simulink model "Final_Model"  (R2018a)
settings: Solver=ode23tb  StartTime=0.0  StopTime=0.15  MaxStep=1e-2  RelTol=1e-3
undefined symbols (not defined in the file): rvar
libraries: powerlib x75, powerlib_extras x4, sps_avr x2, powerlib_meascontrol x1
settings Model: Creator=Mahdi  LastModifiedBy=Lenovo
settings SolverCC: ZeroCrossAlgorithm=Adaptive  SolverResetMethod=Robust
settings DataIOCC: LimitDataPoints=on  SaveFormat=Array
settings OptimizationCC: LifeSpan=inf
settings DebuggingCC: UnderspecifiedInitializationDetection=Classic  MergeDetectMultiDrivingBlocksExec=none  SolverPrmCheckMsg=warning  LibraryContextMissingDiagnostic=warning  SFUnexpectedBacktrackingDiag=warning  SFNoUnconditionalDefaultTransitionDiag=warning  SFExecutionAtInitializationDiag=none
settings HardwareCC: ProdBitPerPointer=32  ProdBitPerSizeT=32  ProdBitPerPtrDiffT=32  ProdLargestAtomicFloat=None  ProdIntDivRoundTo=Undefined  ProdEndianess=Unspecified  ProdWordSize=32  ProdHWDeviceType=32-bit Generic
settings ModelReferenceCC: PropagateSignalLabelsOutOfModel=off
settings CodeAppCC: StateflowObjectComments=on
settings GRTTargetCC: TargetLangStandard=C89/C90 (ANSI)  GeneratePreprocessorConditionals=Disable all
settings ConfigComp: CovMetricSettings=dw  CovHtmlReporting=on  CovSaveCumulativeToWorkspaceVar=on  CovSaveSingleToWorkspaceVar=on  CovExternalEMLEnable=off
settings SimscapeCC: SimscapeNormalizeSystem=off

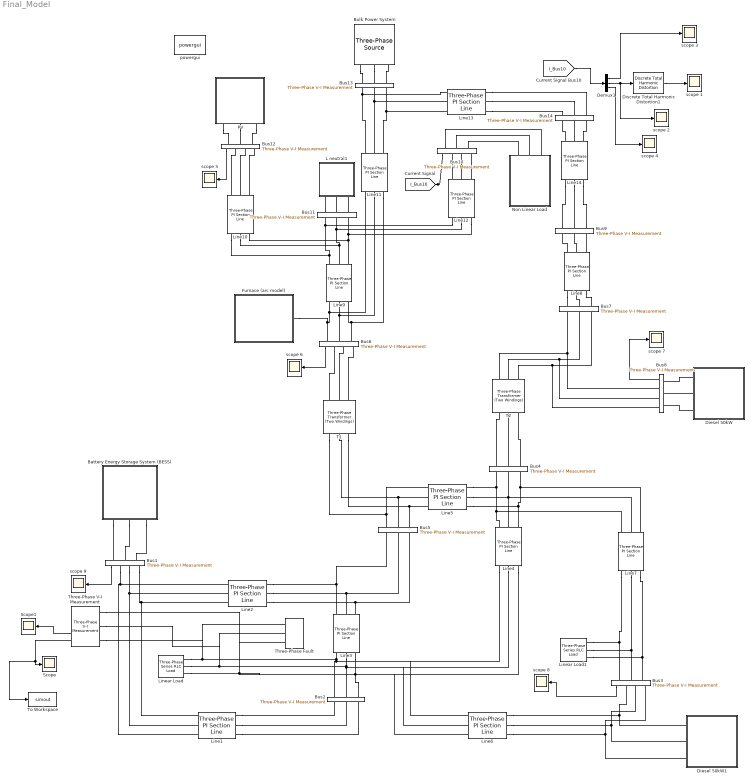
== system Final_Model ==
  " L neutral1" : Subsystem
  Battery Energy Storage System (BESS) : Subsystem
  Bulk Power System : powerlib/Electrical Sources/Three-Phase Source  InternalConnection=Yg  VoltagePhases=off  Voltage=25e3  PhaseAngle=0  Voltage_phases=[25e3 25e3 25e3]/sqrt(3)  PhaseAngles_phases=[0 -120 +120]  Frequency=60  NonIdealSource=on  SpecifyImpedance=on  Resistance=0.8929  Inductance=16.58e-3  ShortCircuitLevel=100e6  BaseVoltage=25e3  XRratio=7  BusType=swing  Pref=0  Qref=0  Prefabc=[10e3, 10e3, 10e3]  Qrefabc=[0, 0, 0]  Qmin=-inf  Qmax=inf
  Bus{1,3,6,8,10,12} (6 alike) : powerlib/Measurements/Three-Phase V-I Measurement  VoltageMeasurement=no  SetLabelV=off  LabelV=Vabc  Vpu=off  VpuLL=off  CurrentMeasurement=yes  SetLabelI=off  LabelI=Iabc  Ipu=off  Pbase=100e6  Vbase=500e3  OutputType=Complex  PhasorSimulation=off  PSBequivalent=0
  Bus{2,4..5,7,9,11,13..14} (8 alike) : powerlib/Measurements/Three-Phase V-I Measurement  VoltageMeasurement=no  SetLabelV=off  LabelV=Vabc  Vpu=off  VpuLL=off  CurrentMeasurement=no  SetLabelI=off  LabelI=Iabc  Ipu=off  Pbase=100e6  Vbase=500e3  OutputType=Complex  PhasorSimulation=off  PSBequivalent=0
  Demux1 : Demux  Outputs=3
  Diesel 50kW : Subsystem
  Diesel 50kW1 : Subsystem
  Discrete Total Harmonic Distortion1 : powerlib_extras/Discrete Measurements/Discrete Total Harmonic Distortion  Freq=50  Ts=50e-6
  Furnace (arc model) : Subsystem
  Line1 : powerlib/Elements/Three-Phase PI Section Line  LConnTagsString=a|b|c  RConnTagsString=A|B|C  Frequency=60  Resistances=[ 0.01273 0.3864]  Inductances="[ 0.9337e-3  4.1264e-3]"  Capacitances=[12.74e-9 7.751e-9]  Length=3
      settings: SourceProductName=Simscape Power Systems
  Line{2..3,6,9..10,12} (6 alike) : powerlib/Elements/Three-Phase PI Section Line  LConnTagsString=a|b|c  RConnTagsString=A|B|C  Frequency=60  Resistances=[ 0.01273 0.3864]  Inductances="[ 0.9337e-3  4.1264e-3]"  Capacitances=[12.74e-9 7.751e-9]  Length=2
      settings: SourceProductName=Simscape Power Systems
  Line11 : powerlib/Elements/Three-Phase PI Section Line  LConnTagsString=a|b|c  RConnTagsString=A|B|C  Frequency=60  Resistances=[ 0.01273 0.3864]  Inductances="[ 0.9337e-3  4.1264e-3]"  Capacitances=[12.74e-9 7.751e-9]  Length=1.5
      settings: SourceProductName=Simscape Power Systems
  Line13 : powerlib/Elements/Three-Phase PI Section Line  LConnTagsString=a|b|c  RConnTagsString=A|B|C  Frequency=60  Resistances=[ 0.01273 0.3864]  Inductances="[ 0.9337e-3  4.1264e-3]"  Capacitances=[12.74e-9 7.751e-9]  Length=1
      settings: SourceProductName=Simscape Power Systems
  Line14 : powerlib/Elements/Three-Phase PI Section Line  LConnTagsString=a|b|c  RConnTagsString=A|B|C  Frequency=60  Resistances=[ 0.01273 0.3864]  Inductances="[ 0.9337e-3  4.1264e-3]"  Capacitances=[12.74e-9 7.751e-9]  Length=1
      settings: SourceProductName=Simscape Power Systems
  Line4 : powerlib/Elements/Three-Phase PI Section Line  LConnTagsString=a|b|c  RConnTagsString=A|B|C  Frequency=60  Resistances=[ 0.01273 0.3864]  Inductances="[ 0.9337e-3  4.1264e-3]"  Capacitances=[12.74e-9 7.751e-9]  Length=3
      settings: SourceProductName=Simscape Power Systems
  Line5 : powerlib/Elements/Three-Phase PI Section Line  LConnTagsString=a|b|c  RConnTagsString=A|B|C  Frequency=60  Resistances=[ 0.01273 0.3864]  Inductances="[ 0.9337e-3  4.1264e-3]"  Capacitances=[12.74e-9 7.751e-9]  Length=3
      settings: SourceProductName=Simscape Power Systems
  Line7 : powerlib/Elements/Three-Phase PI Section Line  LConnTagsString=a|b|c  RConnTagsString=A|B|C  Frequency=60  Resistances=[ 0.01273 0.3864]  Inductances="[ 0.9337e-3  4.1264e-3]"  Capacitances=[12.74e-9 7.751e-9]  Length=2.4
      settings: SourceProductName=Simscape Power Systems
  Line8 : powerlib/Elements/Three-Phase PI Section Line  LConnTagsString=a|b|c  RConnTagsString=A|B|C  Frequency=60  Resistances=[ 0.01273 0.3864]  Inductances="[ 0.9337e-3  4.1264e-3]"  Capacitances=[12.74e-9 7.751e-9]  Length=1
      settings: SourceProductName=Simscape Power Systems
  Linear Load : powerlib/Elements/Three-Phase Series RLC Load  LConnTagsString=A|B|C  Configuration=Y (grounded)  NominalVoltage=1000  Vabc=[1e3 1e3 1e3]  Vabcp=[1e3 1e3 1e3]  NominalFrequency=60  UnbalancedPower=off  ActivePower=1e3  InductivePower=100  CapacitivePower=100  Pabc=[10e3 9e3 11e3]  QLabc=[100 90 110]  QCabc=[100 90 110]  Pabcp=[10e3 9e3 11e3]  QLabcp=[100 90 110]  QCabcp=[100 90 110]  Measurements=None  LoadType=constant Z
  Linear Load1 : powerlib/Elements/Three-Phase Series RLC Load  LConnTagsString=A|B|C  Configuration=Y (grounded)  NominalVoltage=1000  Vabc=[1e3 1e3 1e3]  Vabcp=[1e3 1e3 1e3]  NominalFrequency=60  UnbalancedPower=off  ActivePower=1e3  InductivePower=100  CapacitivePower=100  Pabc=[10e3 9e3 11e3]  QLabc=[100 90 110]  QCabc=[100 90 110]  Pabcp=[10e3 9e3 11e3]  QLabcp=[100 90 110]  QCabcp=[100 90 110]  Measurements=None  LoadType=constant Z
  Non Linear Load : Subsystem
  PV : Subsystem
  Scope : Scope
  Scope1 : Scope
  T1 : powerlib/Elements/Three-Phase Transformer (Two Windings)  Winding1Connection=Yg  Winding2Connection=Yg  CoreType=Three single-phase transformers  SetSaturation=off  Hysteresis=off  DataFile='hysteresis'  SetInitialFlux=off  Measurements=None  UNITS=pu  NominalPower=[ 250e6 , 60 ]  Winding1=[ 0.735e3 , 0.002 , 0.08 ]  Winding2=[ 255e3 , 0.002 , 0.08 ]  Rm=500  Lm=500  L0=0.5  Saturation=[ 0,0 ; 0.0024,1.2 ; 1.0,1.52 ]  InitialFluxes=[ 0.8 , -0.8 , 0.7 ]  MoreParameters=off  BreakLoop=off  DataType=off  TransfoNumber=1
  T2 : powerlib/Elements/Three-Phase Transformer (Two Windings)  Winding1Connection=Yg  Winding2Connection=Yg  CoreType=Three single-phase transformers  SetSaturation=off  Hysteresis=off  DataFile='hysteresis'  SetInitialFlux=off  Measurements=None  UNITS=pu  NominalPower=[ 250e6 , 60 ]  Winding1=[ 0.735e3 , 0.002 , 0.08 ]  Winding2=[ 25e3 , 0.002 , 0.08 ]  Rm=500  Lm=500  L0=0.5  Saturation=[ 0,0 ; 0.0024,1.2 ; 1.0,1.52 ]  InitialFluxes=[ 0.8 , -0.8 , 0.7 ]  MoreParameters=off  BreakLoop=off  DataType=off  TransfoNumber=1
  Three-Phase V-I Measurement : powerlib/Measurements/Three-Phase V-I Measurement  VoltageMeasurement=phase-to-ground  SetLabelV=off  LabelV=Vabc  Vpu=off  VpuLL=off  CurrentMeasurement=yes  SetLabelI=off  LabelI=Iabc  Ipu=off  Pbase=100e6  Vbase=500e3  OutputType=Complex  PhasorSimulation=off  PSBequivalent=0
  Three-Phase Fault : powerlib/Elements/Three-Phase Fault  InitialStates=0  FaultA=on  FaultB=on  FaultC=off  GroundFault=on  SwitchTimes="[0.04  0.08]"  External=off  SwitchStatus=NaN  FaultResistance=0.00001  GroundResistance=0.0001  SnubberResistance=1e6  SnubberCapacitance=inf  Measurements=None
  To Workspace : ToWorkspace  VariableName=simout  SampleTime=-1
  powergui : powerlib/powergui  Priority=1  SimulationMode=Discrete  SampleTime=2e-5  frequency=60  Iterations=50  frequencyindice=0  Pbase=100e6  ErrMax=1e-4  UnitsV=kV  UnitsW=MW  buscounter=0  FunctionMessages=off  echomessages=off  EnableUseOfTLC=off  CurrentSourceSwitches=off  DisableSnubberDevices=off  DisableRonSwitches=off  DisableVfSwitches=off  DisplayEquations=off  SolverType=Tustin  Interpol=off  ExternalGateDelay=off  methode=off  Ts=0  x0status=blocks  SPID=off  SwTol=0  HookPort=off  RestoreLinks=warning  ResistiveCurrentMeasurement=off  Frange=[0:2:500]  Ylog=off  Xlog=on  ShowGrid=off  save=off  variable=ZData  structure=0  ZoomFFT=off  StartTime=0.0  cycles=1  DisplayStyle=1  fundamental=60  FreqAxis=off  MaxFrequency=1000  frequencyindicesteady=1  RmsSteady=1  display=off
  scope {1..9} (9 alike) : Scope
  tag scope: I_Bus10=global
  wires:
  [I_Bus10] -> Demux1/1
  Discrete Total Harmonic Distortion1/1 -> scope 1/1
  Bus10/1 -> [I_Bus10]
  Demux1/2 -> scope 2/1, Discrete Total Harmonic Distortion1/1
  Demux1/1 -> scope 3/1
  Demux1/3 -> scope 4/1
  Bus12/1 -> scope 5/1
  Bus6/1 -> scope 6/1
  Bus8/1 -> scope 7/1
  Bus3/1 -> scope 8/1
  Bus1/1 -> scope 9/1
  Three-Phase V-I Measurement/1 -> To Workspace/1, Scope/1
  Three-Phase V-I Measurement/2 -> Scope1/1
  connections:
  Bus1/RConn1 -- Line1/LConn3 -- Line2/LConn1
  Bus1/RConn2 -- Line1/LConn2 -- Line2/LConn2
  Bus1/RConn3 -- Line1/LConn1 -- Line2/LConn3
  Line1/RConn1 -- Bus2/RConn1
  Line1/RConn2 -- Bus2/RConn2
  Line1/RConn3 -- Bus2/RConn3
  Line2/RConn1 -- Line3/RConn1 -- Bus5/RConn1
  Line2/RConn2 -- Line3/RConn2 -- Bus5/RConn2
  Line2/RConn3 -- Line3/RConn3 -- Bus5/RConn3
  Line3/LConn1 -- Three-Phase Fault/LConn1 -- Three-Phase V-I Measurement/LConn1 -- Linear Load/LConn1 -- Bus2/LConn1 -- Line6/LConn1 -- Line4/LConn1
  Line3/LConn2 -- Three-Phase Fault/LConn2 -- Three-Phase V-I Measurement/LConn2 -- Linear Load/LConn2 -- Line6/LConn2 -- Line4/LConn2 -- Bus2/LConn2
  Line3/LConn3 -- Three-Phase V-I Measurement/LConn3 -- Three-Phase Fault/LConn3 -- Linear Load/LConn3 -- Line6/LConn3 -- Line4/LConn3 -- Bus2/LConn3
  Line4/RConn1 -- Line7/RConn1 -- Bus4/RConn1 -- Line5/RConn1
  Line4/RConn2 -- Line7/RConn2 -- Bus4/RConn2 -- Line5/RConn2
  Line4/RConn3 -- Line5/RConn3 -- Line7/RConn3 -- Bus4/RConn3
  Line5/LConn1 -- T1/LConn1 -- Bus5/LConn1
  Line5/LConn2 -- Bus5/LConn2 -- T1/LConn2
  Line5/LConn3 -- T1/LConn3 -- Bus5/LConn3
  Line6/RConn1 -- Bus3/RConn1 -- Diesel 50kW1/LConn1
  Line6/RConn2 -- Bus3/RConn2 -- Diesel 50kW1/LConn2
  Line6/RConn3 -- Bus3/RConn3 -- Diesel 50kW1/LConn3
  Line7/LConn1 -- Bus3/LConn1 -- Linear Load1/LConn1
  Line7/LConn2 -- Bus3/LConn2 -- Linear Load1/LConn2
  Line7/LConn3 -- Bus3/LConn3 -- Linear Load1/LConn3
  Line8/LConn1 -- Bus7/LConn1
  Bus7/LConn2 -- Line8/LConn2
  Line8/LConn3 -- Bus7/LConn3
  Line8/RConn1 -- Bus9/RConn1
  Line8/RConn2 -- Bus9/RConn2
  Line8/RConn3 -- Bus9/RConn3
  Bus12/RConn1 -- Line10/RConn1
  Bus12/RConn2 -- Line10/RConn2
  Bus12/RConn3 -- Line10/RConn3
  Bus6/LConn1 -- Furnace (arc model)/LConn1 -- Line11/LConn1 -- Line9/LConn1
  Bus6/LConn2 -- Line11/LConn2 -- Line9/LConn2
  Bus6/LConn3 -- Line9/LConn3 -- Line11/LConn3
  Line9/RConn1 -- Line10/LConn1 -- Line12/LConn1 -- Bus11/RConn1
  Line9/RConn2 -- Line10/LConn2 -- Line12/LConn2 -- Bus11/RConn2
  Line9/RConn3 -- Line10/LConn3 -- Line12/LConn3 -- Bus11/RConn3
  Line11/RConn1 -- Line13/LConn1 -- Bus13/RConn1
  Line11/RConn2 -- Bus13/RConn2 -- Line13/LConn2
  Line11/RConn3 -- Bus13/RConn3 -- Line13/LConn3
  Line12/RConn1 -- Bus10/RConn1
  Line12/RConn2 -- Bus10/RConn2
  Line12/RConn3 -- Bus10/RConn3
  Line13/RConn1 -- Bus14/LConn3
  Line13/RConn2 -- Bus14/LConn2
  Line13/RConn3 -- Bus14/LConn1
  Line14/RConn3 -- Bus14/RConn3
  Line14/RConn2 -- Bus14/RConn2
  Line14/RConn1 -- Bus14/RConn1
  Line14/LConn3 -- Bus9/LConn3
  Line14/LConn2 -- Bus9/LConn2
  Line14/LConn1 -- Bus9/LConn1
  T1/RConn1 -- Bus6/RConn1
  T1/RConn2 -- Bus6/RConn2
  T1/RConn3 -- Bus6/RConn3
  Bus4/LConn1 -- T2/LConn1
  Bus4/LConn2 -- T2/LConn2
  Bus4/LConn3 -- T2/LConn3
  T2/RConn1 -- Bus8/RConn1 -- Bus7/RConn1
  T2/RConn2 -- Bus8/RConn2 -- Bus7/RConn2
  T2/RConn3 -- Bus8/RConn3 -- Bus7/RConn3
  Diesel 50kW/LConn1 -- Bus8/LConn1
  Diesel 50kW/LConn2 -- Bus8/LConn2
  Diesel 50kW/LConn3 -- Bus8/LConn3
  Battery Energy Storage System (BESS)/LConn1 -- Bus1/LConn1
  Battery Energy Storage System (BESS)/LConn2 -- Bus1/LConn2
  Battery Energy Storage System (BESS)/LConn3 -- Bus1/LConn3
  PV/LConn1 -- Bus12/LConn1
  PV/LConn2 -- Bus12/LConn2
  PV/LConn3 -- Bus12/LConn3
  Bus11/LConn1 -- " L neutral1"/LConn1
  Bus11/LConn2 -- " L neutral1"/LConn2
  Bus11/LConn3 -- " L neutral1"/LConn3
  Non Linear Load/LConn1 -- Bus10/LConn3
  Non Linear Load/LConn2 -- Bus10/LConn2
  Non Linear Load/LConn3 -- Bus10/LConn1
  Bulk Power System/RConn1 -- Bus13/LConn1
  Bulk Power System/RConn2 -- Bus13/LConn2
  Bulk Power System/RConn3 -- Bus13/LConn3

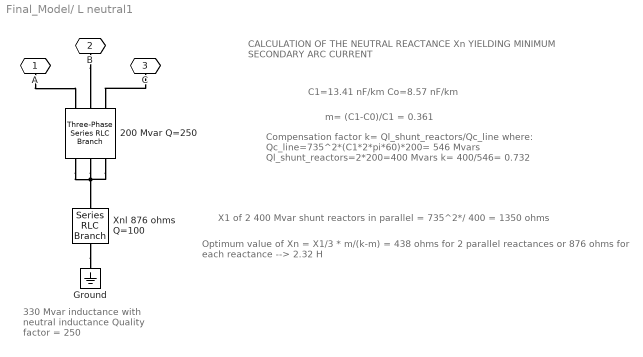
== system Final_Model/ L neutral1 ==
  note: CALCULATION OF THE NEUTRAL REACTANCE Xn
      | YIELDING MINIMUM SECONDARY ARC CURRENT
  note: X1 of 2 400 Mvar shunt reactors in parallel = 735^2*/ 400 = 1350 ohms
  note: Optimum value of Xn = X1/3 * m/(k-m) = 438 ohms for 2 parallel reactances
      | or 876 ohms for each reactance --> 2.32 H
  note: Compensation factor k= Ql_shunt_reactors/Qc_line
      | where:
      |  Qc_line=735^2*(C1*2*pi*60)*200= 546 Mvars
      |  Ql_shunt_reactors=2*200=400 Mvars
      | k= 400/546= 0.732
  note: m= (C1-C0)/C1 = 0.361
  note: C1=13.41 nF/km Co=8.57 nF/km
  note: 330 Mvar inductance
      | with neutral inductance
      | Quality factor = 250
  200 Mvar Q=250 : powerlib/Elements/Three-Phase Series RLC Branch  LConnTagsString=A|B|C  RConnTagsString=A|B|C  BranchType=RL  Resistance=735^2/200/250  Inductance=.735^2/.200/.377  Capacitance=1.0  Measurements=None
  Ground : powerlib/Elements/Ground  LConnTagsString=a
  Xnl 876 ohms Q=100 : powerlib/Elements/Series RLC Branch  LConnTagsString=__new0  RConnTagsString=__new0  BranchType=RL  Resistance=876/100  Inductance=8.76/377  SetiL0=off  InitialCurrent=0  Capacitance=1.0  Setx0=off  InitialVoltage=0  Measurements=None
  A : PMIOPort  Side=Left
  B : PMIOPort  Port=2  Side=Left
  C : PMIOPort  Port=3  Side=Left
  connections:
  A/RConn1 -- 200 Mvar Q=250/LConn1
  B/RConn1 -- 200 Mvar Q=250/LConn2
  C/RConn1 -- 200 Mvar Q=250/LConn3
  200 Mvar Q=250/RConn3 -- 200 Mvar Q=250/RConn2 -- Xnl 876 ohms Q=100/LConn1 -- 200 Mvar Q=250/RConn1
  Xnl 876 ohms Q=100/RConn1 -- Ground/LConn1

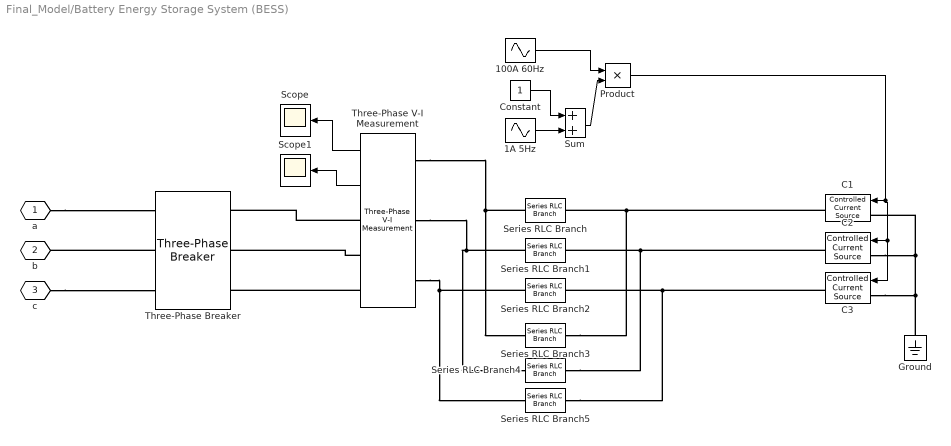
== system Final_Model/Battery Energy Storage System (BESS) ==
  100A 60Hz : Sin  Amplitude=100  Frequency=2*pi*60  SampleTime=0
  1A 5Hz : Sin  Frequency=2*pi*5  SampleTime=0
  C1 : powerlib/Electrical Sources/Controlled Current Source  Initialize=on  Source_Type=AC  Amplitude=0  Phase=0  Frequency=0  Measurements=None
  C2 : powerlib/Electrical Sources/Controlled Current Source  Initialize=on  Source_Type=AC  Amplitude=0  Phase=0  Frequency=0  Measurements=None
  C3 : powerlib/Electrical Sources/Controlled Current Source  Initialize=on  Source_Type=AC  Amplitude=0  Phase=0  Frequency=0  Measurements=None
  Constant : Constant
  Ground : powerlib/Elements/Ground  LConnTagsString=a
  Product : Product  SaturateOnIntegerOverflow=on  InputSameDT=on  OutDataTypeStr=Inherit: Same as first input
  Scope : Scope
  Scope1 : Scope
  Series RLC Branch : powerlib/Elements/Series RLC Branch  LConnTagsString=__new0  RConnTagsString=__new0  BranchType=L  Resistance=1  Inductance=1e-3  SetiL0=off  InitialCurrent=0  Capacitance=1e-6  Setx0=off  InitialVoltage=0  Measurements=None
  Series RLC Branch1 : powerlib/Elements/Series RLC Branch  LConnTagsString=__new0  RConnTagsString=__new0  BranchType=L  Resistance=1  Inductance=1e-3  SetiL0=off  InitialCurrent=0  Capacitance=1e-6  Setx0=off  InitialVoltage=0  Measurements=None
  Series RLC Branch2 : powerlib/Elements/Series RLC Branch  LConnTagsString=__new0  RConnTagsString=__new0  BranchType=L  Resistance=1  Inductance=1e-3  SetiL0=off  InitialCurrent=0  Capacitance=1e-6  Setx0=off  InitialVoltage=0  Measurements=None
  Series RLC Branch3 : powerlib/Elements/Series RLC Branch  LConnTagsString=__new0  RConnTagsString=__new0  BranchType=R  Resistance=1  Inductance=1e-3  SetiL0=off  InitialCurrent=0  Capacitance=1e-6  Setx0=off  InitialVoltage=0  Measurements=None
  Series RLC Branch4 : powerlib/Elements/Series RLC Branch  LConnTagsString=__new0  RConnTagsString=__new0  BranchType=R  Resistance=1  Inductance=1e-3  SetiL0=off  InitialCurrent=0  Capacitance=1e-6  Setx0=off  InitialVoltage=0  Measurements=None
  Series RLC Branch5 : powerlib/Elements/Series RLC Branch  LConnTagsString=__new0  RConnTagsString=__new0  BranchType=R  Resistance=1  Inductance=1e-3  SetiL0=off  InitialCurrent=0  Capacitance=1e-6  Setx0=off  InitialVoltage=0  Measurements=None
  Sum : Sum  SaturateOnIntegerOverflow=on  InputSameDT=on  OutDataTypeStr=Inherit: Same as first input
  Three-Phase V-I Measurement : powerlib/Measurements/Three-Phase V-I Measurement  VoltageMeasurement=phase-to-ground  SetLabelV=off  LabelV=Vabc  Vpu=off  VpuLL=off  CurrentMeasurement=yes  SetLabelI=off  LabelI=Iabc  Ipu=off  Pbase=100e6  Vbase=500e3  OutputType=Complex  PhasorSimulation=off  PSBequivalent=0
  Three-Phase Breaker : powerlib/Elements/Three-Phase Breaker  InitialState=closed  SwitchA=on  SwitchB=on  SwitchC=on  SwitchTimes="[4/60  10/60]"  External=off  BreakerResistance=0.001  SnubberResistance=1e6  SnubberCapacitance=inf  Measurements=None
  "a " : PMIOPort  Tag=PMCPort  Side=Left
  b : PMIOPort  Tag=PMCPort  Port=2  Side=Left
  c : PMIOPort  Tag=PMCPort  Port=3  Side=Left
  wires:
  1A 5Hz/1 -> Sum/2
  Constant/1 -> Sum/1
  Sum/1 -> Product/2
  100A 60Hz/1 -> Product/1
  Three-Phase V-I Measurement/1 -> Scope/1
  Three-Phase V-I Measurement/2 -> Scope1/1
  Product/1 -> C3/1, C2/1, C1/1
  connections:
  c/RConn1 -- Three-Phase Breaker/LConn3
  "a "/RConn1 -- Three-Phase Breaker/LConn1
  Series RLC Branch1/LConn1 -- Three-Phase V-I Measurement/LConn2 -- Series RLC Branch4/LConn1
  Series RLC Branch/LConn1 -- Series RLC Branch3/LConn1 -- Three-Phase V-I Measurement/LConn1
  Series RLC Branch2/LConn1 -- Three-Phase V-I Measurement/LConn3 -- Series RLC Branch5/LConn1
  C1/RConn1 -- Series RLC Branch3/RConn1 -- Series RLC Branch/RConn1
  C2/RConn1 -- Series RLC Branch4/RConn1 -- Series RLC Branch1/RConn1
  C3/RConn1 -- Series RLC Branch5/RConn1 -- Series RLC Branch2/RConn1
  Ground/LConn1 -- C3/LConn1 -- C2/LConn1 -- C1/LConn1
  Three-Phase Breaker/LConn2 -- b/RConn1
  Three-Phase V-I Measurement/RConn3 -- Three-Phase Breaker/RConn3
  Three-Phase V-I Measurement/RConn2 -- Three-Phase Breaker/RConn2
  Three-Phase V-I Measurement/RConn1 -- Three-Phase Breaker/RConn1

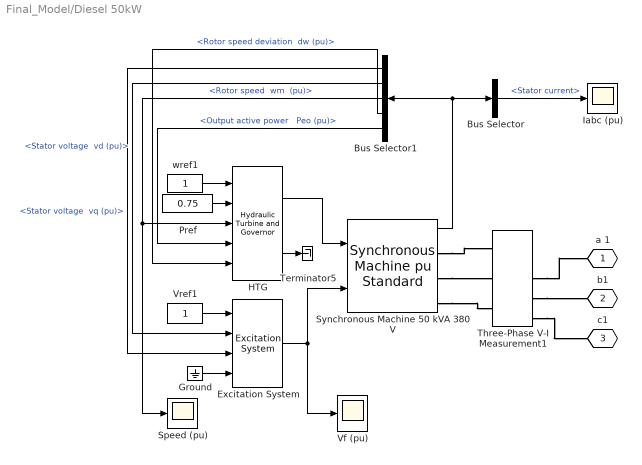
== system Final_Model/Diesel 50kW ==
  " Iabc (pu)" : Scope
  " Speed (pu)" : Scope
  Bus Selector : BusSelector  OutputSignals=Stator current
  Bus Selector1 : BusSelector  OutputSignals="dq0 components.Stator voltage  vq (pu),dq0 components.Stator voltage  vd (pu),Mechanical.Rotor speed  wm  (pu),Mechanical.Rotor speed deviation  dw (pu),Output active power   Peo (pu)"
  Excitation System : sps_avr/Excitation System  tr=20e-3  reg=[ 300, 0.001 ]  exc=[ 1, 0 ]  tgr=[ 0, 0 ]  damp=[ 0.001, 0.1 ]  sat=[ 0, 0 ]  lim=[ -11.5, 11.5, 0 ]  v0=[1,1.29071]
      settings: SourceProductName=Simscape Power Systems  SourceProductBaseCode=PS
  Ground : Ground
  HTG : powerlib/Machines/Hydraulic Turbine and Governor  sm="[ 10/3  0.07 ]"  gate="[  0.01  0.97518  -0.1  0.1 ]"  reg="[  0.05  1.163  0.105  0  0.01  ]"  hyd="[  0  2.67  ]"  dref=0  po=0.751606
      settings: SourceProductName=Simscape Power Systems  SourceProductBaseCode=PS
  Pref : Constant  Value=0.75
  Synchronous Machine 50 kVA 380 V : powerlib/Machines/Synchronous Machine pu Standard  PresetModel=No  MechanicalLoad=Mechanical power Pm  ShowDetailedParameters=on  RotorType=Salient-pole  Units=per unit standard parameters  MeasurementBus=off  NominalParameters="[ 50E3  380   60 ]"  Reactances1=[ 31 32 33 34 35 36 37 ]  Reactances2=[ 1.305, 0.296, 0.252, 0.474, 0.243, 0.18 ]  dAxisTimeConstants=Short-circuit  qAxisTimeConstants=Open-circuit  TimeConstants1=[]  TimeConstants2=[]  TimeConstants3=[]  TimeConstants4=[]  TimeConstants5=[ 1.01, 0.053, 0.1 ]  TimeConstants6=[]  TimeConstants7=[]  TimeConstants8=[]  StatorResistance=2.8544e-3  Mechanical=[ 3.2 0 2]  PolePairs=2  InitialConditions=[0 -94.2826 0.750185 0.750185 0.750185 -24.943 -144.943 95.057 1.29071]  SetSaturation=off  Saturation=[0.6404,0.7127,0.8441,0.9214,0.9956,1.082,1.19,1.316,1.457;0.7,0.7698,0.8872,0.9466,0.9969,1.046,1.1,1.151,1.201]  LoadFlowParameters=[1 150000000 0 0]  TsPowergui=0  TsBlock=-1  IterativeModel=Trapezoidal iterative (alg. loop)  IterativeDiscreteModel=Trapezoidal non iterative  BusType=PV  Pref=150000000  Qref=0  Qmin=-Inf  Qmax=Inf  PLF=0  QLF=0
      settings: AttributesFormatString=\n\n  SourceProductName=Simscape Power Systems
  Terminator5 : Terminator
  Three-Phase V-I Measurement1 : powerlib/Measurements/Three-Phase V-I Measurement  VoltageMeasurement=phase-to-ground  SetLabelV=off  LabelV=Vabc  Vpu=off  VpuLL=off  CurrentMeasurement=yes  SetLabelI=off  LabelI=Iabc  Ipu=off  Pbase=100e6  Vbase=500e3  OutputType=Complex  PhasorSimulation=off  PSBequivalent=0
  Vf (pu) : Scope
  Vref1 : Constant
  wref1 : Constant
  a 1 : PMIOPort  Tag=PMCPort  Side=Left
  b1 : PMIOPort  Tag=PMCPort  Port=2  Side=Left
  c1 : PMIOPort  Tag=PMCPort  Port=3  Side=Left
  wires:
  Ground/1 -> Excitation System/4
  HTG/2 -> Terminator5/1
  Pref/1 -> HTG/2
  Excitation System/1 -> Vf (pu)/1, Synchronous Machine 50 kVA 380 V/2
  HTG/1 -> Synchronous Machine 50 kVA 380 V/1
  Synchronous Machine 50 kVA 380 V/1 -> Bus Selector/1, Bus Selector1/1
  Bus Selector/1 -> " Iabc (pu)"/1  "<Stator current>"
  Bus Selector1/1 -> Excitation System/3  "<Stator voltage  vq (pu)>"
  Bus Selector1/2 -> Excitation System/2  "<Stator voltage  vd (pu)>"
  Bus Selector1/3 -> HTG/3, " Speed (pu)"/1  "<Rotor speed  wm  (pu)>"
  Bus Selector1/4 -> HTG/5  "<Rotor speed deviation  dw (pu)>"
  Bus Selector1/5 -> HTG/4  "<Output active power   Peo (pu)>"
  Vref1/1 -> Excitation System/1
  wref1/1 -> HTG/1
  connections:
  Synchronous Machine 50 kVA 380 V/RConn1 -- Three-Phase V-I Measurement1/LConn1
  Synchronous Machine 50 kVA 380 V/RConn2 -- Three-Phase V-I Measurement1/LConn2
  Synchronous Machine 50 kVA 380 V/RConn3 -- Three-Phase V-I Measurement1/LConn3
  Three-Phase V-I Measurement1/RConn1 -- a 1/RConn1
  Three-Phase V-I Measurement1/RConn2 -- b1/RConn1
  Three-Phase V-I Measurement1/RConn3 -- c1/RConn1

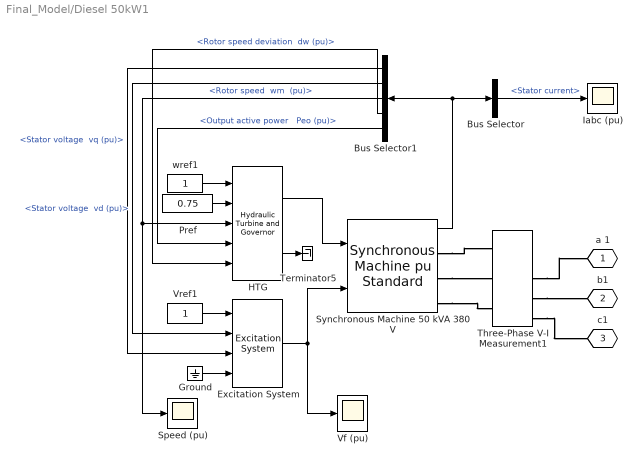
== system Final_Model/Diesel 50kW1 ==
  " Iabc (pu)" : Scope
  " Speed (pu)" : Scope
  Bus Selector : BusSelector  OutputSignals=Stator current
  Bus Selector1 : BusSelector  OutputSignals="dq0 components.Stator voltage  vq (pu),dq0 components.Stator voltage  vd (pu),Mechanical.Rotor speed  wm  (pu),Mechanical.Rotor speed deviation  dw (pu),Output active power   Peo (pu)"
  Excitation System : sps_avr/Excitation System  tr=20e-3  reg=[ 300, 0.001 ]  exc=[ 1, 0 ]  tgr=[ 0, 0 ]  damp=[ 0.001, 0.1 ]  sat=[ 0, 0 ]  lim=[ -11.5, 11.5, 0 ]  v0=[1,1.29071]
      settings: SourceProductName=Simscape Power Systems  SourceProductBaseCode=PS
  Ground : Ground
  HTG : powerlib/Machines/Hydraulic Turbine and Governor  sm="[ 10/3  0.07 ]"  gate="[  0.01  0.97518  -0.1  0.1 ]"  reg="[  0.05  1.163  0.105  0  0.01  ]"  hyd="[  0  2.67  ]"  dref=0  po=0.751606
      settings: SourceProductName=Simscape Power Systems  SourceProductBaseCode=PS
  Pref : Constant  Value=0.75
  Synchronous Machine 50 kVA 380 V : powerlib/Machines/Synchronous Machine pu Standard  PresetModel=No  MechanicalLoad=Mechanical power Pm  ShowDetailedParameters=on  RotorType=Salient-pole  Units=per unit standard parameters  MeasurementBus=off  NominalParameters="[ 50E3  380   60 ]"  Reactances1=[ 31 32 33 34 35 36 37 ]  Reactances2=[ 1.305, 0.296, 0.252, 0.474, 0.243, 0.18 ]  dAxisTimeConstants=Short-circuit  qAxisTimeConstants=Open-circuit  TimeConstants1=[]  TimeConstants2=[]  TimeConstants3=[]  TimeConstants4=[]  TimeConstants5=[ 1.01, 0.053, 0.1 ]  TimeConstants6=[]  TimeConstants7=[]  TimeConstants8=[]  StatorResistance=2.8544e-3  Mechanical=[ 3.2 0 2]  PolePairs=2  InitialConditions=[0 -94.2826 0.750185 0.750185 0.750185 -24.943 -144.943 95.057 1.29071]  SetSaturation=off  Saturation=[0.6404,0.7127,0.8441,0.9214,0.9956,1.082,1.19,1.316,1.457;0.7,0.7698,0.8872,0.9466,0.9969,1.046,1.1,1.151,1.201]  LoadFlowParameters=[1 150000000 0 0]  TsPowergui=0  TsBlock=-1  IterativeModel=Trapezoidal iterative (alg. loop)  IterativeDiscreteModel=Trapezoidal non iterative  BusType=PV  Pref=150000000  Qref=0  Qmin=-Inf  Qmax=Inf  PLF=0  QLF=0
      settings: AttributesFormatString=\n\n  SourceProductName=Simscape Power Systems
  Terminator5 : Terminator
  Three-Phase V-I Measurement1 : powerlib/Measurements/Three-Phase V-I Measurement  VoltageMeasurement=phase-to-ground  SetLabelV=off  LabelV=Vabc  Vpu=off  VpuLL=off  CurrentMeasurement=yes  SetLabelI=off  LabelI=Iabc  Ipu=off  Pbase=100e6  Vbase=500e3  OutputType=Complex  PhasorSimulation=off  PSBequivalent=0
  Vf (pu) : Scope
  Vref1 : Constant
  wref1 : Constant
  a 1 : PMIOPort  Tag=PMCPort  Side=Left
  b1 : PMIOPort  Tag=PMCPort  Port=2  Side=Left
  c1 : PMIOPort  Tag=PMCPort  Port=3  Side=Left
  wires:
  wref1/1 -> HTG/1
  Vref1/1 -> Excitation System/1
  Bus Selector1/5 -> HTG/4  "<Output active power   Peo (pu)>"
  Bus Selector1/4 -> HTG/5  "<Rotor speed deviation  dw (pu)>"
  Bus Selector1/3 -> " Speed (pu)"/1, HTG/3  "<Rotor speed  wm  (pu)>"
  Bus Selector1/2 -> Excitation System/2  "<Stator voltage  vd (pu)>"
  Bus Selector1/1 -> Excitation System/3  "<Stator voltage  vq (pu)>"
  Bus Selector/1 -> " Iabc (pu)"/1  "<Stator current>"
  Synchronous Machine 50 kVA 380 V/1 -> Bus Selector1/1, Bus Selector/1
  HTG/1 -> Synchronous Machine 50 kVA 380 V/1
  Excitation System/1 -> Synchronous Machine 50 kVA 380 V/2, Vf (pu)/1
  Pref/1 -> HTG/2
  HTG/2 -> Terminator5/1
  Ground/1 -> Excitation System/4
  connections:
  Three-Phase V-I Measurement1/RConn3 -- c1/RConn1
  Three-Phase V-I Measurement1/RConn2 -- b1/RConn1
  Three-Phase V-I Measurement1/RConn1 -- a 1/RConn1
  Synchronous Machine 50 kVA 380 V/RConn3 -- Three-Phase V-I Measurement1/LConn3
  Synchronous Machine 50 kVA 380 V/RConn2 -- Three-Phase V-I Measurement1/LConn2
  Synchronous Machine 50 kVA 380 V/RConn1 -- Three-Phase V-I Measurement1/LConn1

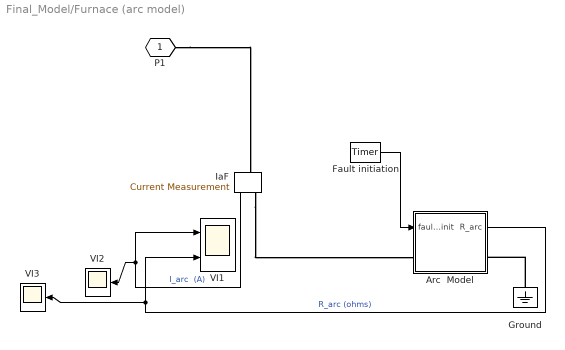
== system Final_Model/Furnace (arc model) ==
  Arc  Model : Subsystem  mask(Arc model){Rarc_var=on, Rarc_fixed=0.1, Rparam=[56.54 0.006375], I0=50, Ts=50e-6}
      mask prompts: Rarc_var "Variable arc resistance :"; Rarc_fixed "Arc resistance for fixed arc resistance :"; Rparam "Arc parameters for variable arc resistance [Ro k] : :"; I0 "Current threshold for arc extinction Io (A rms) :"; Ts "Sample time (s) :"
      mask help:
      | This block implements a variable or fixed arc resistance model.
      |
      | Input 1, output 1:  Connection terminals of the arc resistance.
      | Input 2 :    Control signal for the fault initiation
      | Use a short pulse of 1 cycle. Once fault current starts flowing, it is sustained by the arc ionized path.
      | Output 2:  Arc resitance
      |
      | If you check the 'Variable arc resistance' box, the mean arc resistance will be a function of the arc current, according to equation below. Otherwise, the resistance will be kept constant.
      |
      |        Rarc= Ro*exp(-k*i)
      |
      | where:   i = rms value of the arc current (A)
      |              Ro, k = arc parameters
      |
      | The arc extinguishes at the next zero current crossing after its  rms value has fallen  below  the specified threshold current Io.
      mask init:
      | if strcmp(Rarc_var,'on'), rvar=1; else, rvar=0; end
      | R0=Rparam(1);
      | k=Rparam(2);
  Fault initiation : powerlib_extras/Control  Blocks/Timer  t=[ 1/60 2/60 ]  e="[1 0  ]"
  Ground : powerlib/Elements/Ground  LConnTagsString=a
  IaF : powerlib/Measurements/Current Measurement  Tag=PoWeRsYsTeMmEaSuReMeNt  PhasorSimulation=off  OutputType=Magnitude  PSBequivalent=0
  VI1 : Scope  NumInputPorts=2
  VI2 : Scope
  VI3 : Scope
  P1 : PMIOPort  Tag=PMCPort  Side=Left
  wires:
  Fault initiation/1 -> Arc  Model/1(fault_init)
  Arc  Model/1(R_arc) -> VI1/2, VI3/1  "R_arc (ohms)"
  IaF/1 -> VI1/1, VI2/1  "I_arc  (A)"
  connections:
  Ground/LConn1 -- Arc  Model/RConn1
  IaF/RConn1 -- Arc  Model/LConn1
  P1/RConn1 -- IaF/LConn1

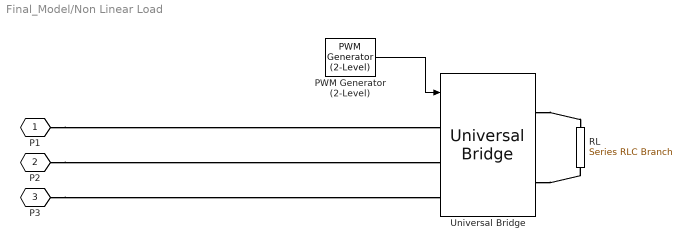
== system Final_Model/Non Linear Load ==
  PWM Generator (2-Level) : powerlib_meascontrol/Pulse & Signal Generators/PWM Generator (2-Level)  ModulatorType=Three-phase bridge (6 pulses)  ModulatorMode=Unsynchronized  Fc=4080  Pc=90  nF=27  MinMax="[ -1  1 ]"  SamplingTechnique=Natural  ModulatingSignals=on  m=0.8  Freq=60  Phase=0  Ts=0  ShowCarrierOutport=off
      settings: SourceProductName=Simscape Power Systems
  RL : powerlib/Elements/Series RLC Branch  LConnTagsString=__new0  RConnTagsString=__new0  BranchType=RL  Resistance=1  Inductance=5e-3  SetiL0=off  InitialCurrent=0  Capacitance=1e-6  Setx0=off  InitialVoltage=0  Measurements=None
  Universal Bridge : powerlib/Power Electronics/Universal Bridge  Arms=3  SnubberResistance=1e5  SnubberCapacitance=inf  Device=Thyristors  Ron=1e-3  Lon=0  ForwardVoltages="[  0  0  ]"  ForwardVoltage=0  GTOparameters=[ 10e-6 , 20e-6 ]  IGBTparameters=[ 1e-6 , 2e-6 ]  Measurements=None  Measurements_2=None  converterType=Rectifier
  P1 : PMIOPort  Tag=PMCPort  Side=Left
  P2 : PMIOPort  Tag=PMCPort  Port=2  Side=Left
  P3 : PMIOPort  Tag=PMCPort  Port=3  Side=Left
  wires:
  PWM Generator (2-Level)/1 -> Universal Bridge/1
  connections:
  Universal Bridge/RConn1 -- RL/LConn1
  P1/RConn1 -- Universal Bridge/LConn1
  P3/RConn1 -- Universal Bridge/LConn3
  P2/RConn1 -- Universal Bridge/LConn2
  Universal Bridge/RConn2 -- RL/RConn1

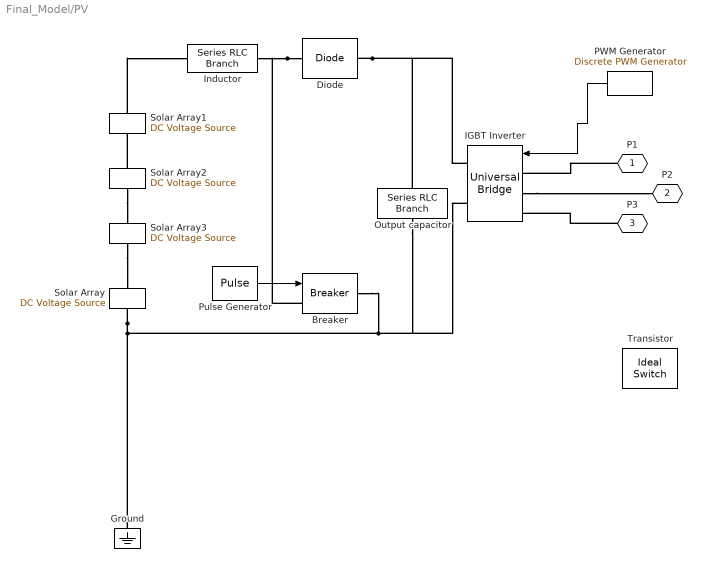
== system Final_Model/PV ==
  Breaker : powerlib/Elements/Breaker  InitialState=0  SwitchingTimes="[ 1/60  5/60 ]"  External=on  BreakerResistance=0.01  SnubberResistance=1e6  SnubberCapacitance=inf  Measurements=None  MoreParameters=off  NoBreakLoop=off
      settings: SourceProductName=Simscape Power Systems
  Diode : powerlib/Power Electronics/Diode  Ron=0.001  Lon=0  Vf=0.8  IC=0  UseSnubber=off  Rs=500  Cs=250e-9  Measurements=off
  Ground : powerlib/Elements/Ground  LConnTagsString=a
  IGBT Inverter : powerlib/Power Electronics/Universal Bridge  Arms=3  SnubberResistance=1e5  SnubberCapacitance=inf  Device=IGBT / Diodes  Ron=1e-3  Lon=0  ForwardVoltages="[  0  0  ]"  ForwardVoltage=0  GTOparameters=[ 10e-6 , 20e-6 ]  IGBTparameters=[ 1e-6 , 2e-6 ]  Measurements=All voltages and currents  Measurements_2=None  converterType=Rectifier
  Inductor : powerlib/Elements/Series RLC Branch  LConnTagsString=__new0  RConnTagsString=__new0  BranchType=L  Resistance=1  Inductance=100e-3  SetiL0=off  InitialCurrent=0  Capacitance=1e-6  Setx0=off  InitialVoltage=0  Measurements=Branch current
  Output capacitor : powerlib/Elements/Series RLC Branch  LConnTagsString=__new0  RConnTagsString=__new0  BranchType=C  Resistance=1.0  Inductance=1e-3  SetiL0=off  InitialCurrent=0  Capacitance=1000e-6  Setx0=off  InitialVoltage=0  Measurements=None
  PWM Generator : powerlib_extras/Discrete  Control Blocks/Discrete PWM Generator  GeneratorMode="3-arm  bridge (6 pulses)"  Fc=900  Ts=5.14e-6  Internal=on  mIndex=0.85  Freq=50  Phase=0
  Pulse Generator : DiscretePulseGenerator  PulseType=Time based  Amplitude=5  Period=1e-6  PulseWidth=50
  Solar Array{,1..3} (4 alike) : powerlib/Electrical Sources/DC Voltage Source  Amplitude=35  Measurements=None
  Transistor : powerlib/Power Electronics/Ideal Switch  Ron=0.001  Lon=0  IC=0  Rs=1e5  Cs=inf  Measurements=on
  "P1 " : PMIOPort  Tag=PMCPort  Side=Left
  P2 : PMIOPort  Tag=PMCPort  Port=2  Side=Left
  P3 : PMIOPort  Tag=PMCPort  Port=3  Side=Left
  wires:
  PWM Generator/1 -> IGBT Inverter/1
  Pulse Generator/1 -> Breaker/1
  connections:
  Solar Array/LConn1 -- Breaker/RConn1 -- IGBT Inverter/RConn2 -- Output capacitor/RConn1 -- Ground/LConn1
  Diode/LConn1 -- Breaker/LConn1 -- Inductor/RConn1
  Diode/RConn1 -- IGBT Inverter/RConn1 -- Output capacitor/LConn1
  Solar Array3/LConn1 -- Solar Array/RConn1
  Solar Array2/RConn1 -- Solar Array1/LConn1
  "P1 "/RConn1 -- IGBT Inverter/LConn1
  P3/RConn1 -- IGBT Inverter/LConn3
  Solar Array2/LConn1 -- Solar Array3/RConn1
  Solar Array1/RConn1 -- Inductor/LConn1
  IGBT Inverter/LConn2 -- P2/RConn1

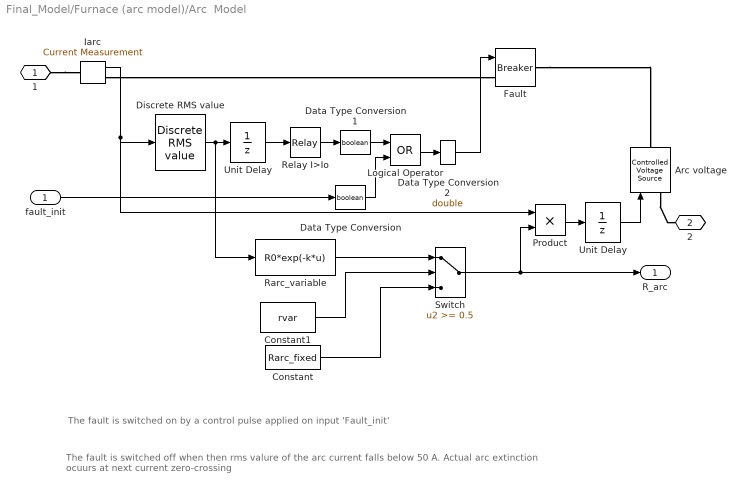
== system Final_Model/Furnace (arc model)/Arc  Model ==
  note: The fault is switched on by a control pulse applied on input 'Fault_init'
  note: The fault is switched off when then rms valure of the arc current falls below  50 A.
      | Actual arc extinction ocuurs at next current zero-crossing
  fault_init : Inport
  Arc voltage : powerlib/Electrical Sources/Controlled Voltage Source  Description=source block  Initialize=on  Source_Type=AC  Amplitude=0  Phase=0  Frequency=0  Measurements=None
      settings: AttributesFormatString=\n
  Constant : Constant  Value=Rarc_fixed
  Constant1 : Constant  Value=rvar
  Data Type Conversion : DataTypeConversion  OutDataTypeStr=boolean  SaturateOnIntegerOverflow=on  RndMeth=Zero
  Data Type Conversion1 : DataTypeConversion  OutDataTypeStr=boolean  SaturateOnIntegerOverflow=on  RndMeth=Zero
  Data Type Conversion2 : DataTypeConversion  OutDataTypeStr=double  SaturateOnIntegerOverflow=on  RndMeth=Zero
  Discrete RMS value : powerlib_extras/Discrete Measurements/Discrete  RMS value  Freq=60  Mag_Init=0  Ts=Ts
  Fault : powerlib/Elements/Breaker  InitialState=0  SwitchingTimes="[ 4/60  5/60 ]"  External=on  BreakerResistance=.001  SnubberResistance=inf  SnubberCapacitance=0  Measurements=None  MoreParameters=off  NoBreakLoop=off
      settings: AttributesFormatString=\n  SourceProductName=Simscape Power Systems
  Iarc : powerlib/Measurements/Current Measurement  Tag=PoWeRsYsTeMmEaSuReMeNt  PhasorSimulation=off  OutputType=Magnitude  PSBequivalent=0
  Logical Operator : Logic  Operator=OR
  Product : Product  SaturateOnIntegerOverflow=on  InputSameDT=on  OutDataTypeStr=Inherit: Same as first input
  Rarc_variable : Fcn  Expr=R0*exp(-k*u)
  Relay I>Io : Relay  OnSwitchValue=I0*1.2  OffSwitchValue=I0  ZeroCross=off
  Switch : Switch  Threshold=0.5  ZeroCross=off  InputSameDT=on
  Unit Delay : UnitDelay  SampleTime=Ts
  "Unit Delay " : UnitDelay  SampleTime=Ts
  1 : PMIOPort  Side=Left
  2 : PMIOPort  Port=2  Side=Right
  R_arc : Outport
  wires:
  Discrete RMS value/1 -> "Unit Delay "/1, Rarc_variable/1
  Rarc_variable/1 -> Switch/1
  Switch/1 -> Product/2, R_arc/1
  Constant/1 -> Switch/3
  Constant1/1 -> Switch/2
  Product/1 -> Unit Delay/1
  "Unit Delay "/1 -> Relay I>Io/1
  fault_init/1 -> Data Type Conversion/1
  Data Type Conversion/1 -> Logical Operator/2
  Relay I>Io/1 -> Data Type Conversion1/1
  Data Type Conversion1/1 -> Logical Operator/1
  Logical Operator/1 -> Data Type Conversion2/1
  Iarc/1 -> Product/1, Discrete RMS value/1
  Unit Delay/1 -> Arc voltage/1
  Data Type Conversion2/1 -> Fault/1
  connections:
  1/RConn1 -- Iarc/LConn1
  Iarc/RConn1 -- Fault/LConn1
  Arc voltage/LConn1 -- 2/RConn1
  Fault/RConn1 -- Arc voltage/RConn1
